simulink model "SimHA"  (R2022a)
settings: Solver=VariableStepAuto  StartTime=0.0  StopTime=20  RelTol=1e-3
values from neighbouring files (symbols this model uses):
  A = [4  0  0; 0  -9  0; 0  0  -1]    [HA1.mat]    (also in HA_1Matlabfile.m = [4 0 0; Home_assignment_1_Matlab_file.m = [4 0 0;0 -9 0;0 0 -1])
  B = [1  0; 1  0; 0  1]    [HA1.mat]    (also in HA_1Matlabfile.m = [1 0; Home_assignment_1_Matlab_file.m = [1 0;1 0;0 1])
  B1 = [1 1 0]    [HA1.mat]    (also in HA_1Matlabfile.m = [1; 1; 0]; Home_assignment_1_Matlab_file.m = [1;1;0])
  B2 = [0 0 1]    [HA1.mat]    (also in HA_1Matlabfile.m = [0; 0; 1]; Home_assignment_1_Matlab_file.m = [0;0;1])
  C = [-8  -9  1; 0  3  -3]    [HA1.mat]    (also in HA_1Matlabfile.m = [-8 -9 1; Home_assignment_1_Matlab_file.m = [-8 -9 1;0 3 -3])
  C1 = [-8 -9 -1]    [HA1.mat]    (also in HA_1Matlabfile.m = [-8 -9 1]; Home_assignment_1_Matlab_file.m)
  C2 = [0 3 -3]    [HA1.mat]    (also in HA_1Matlabfile.m; Home_assignment_1_Matlab_file.m)
  FV1 = [fv1 fv2 0]    [Home_assignment_1_Matlab_file.m]
  FV2 = [0 0 fv3]    [Home_assignment_1_Matlab_file.m]
  V1 = -3.36111388889    [HA1.mat]    (also in Home_assignment_1_Matlab_file.m = inv(-C1*inv(Abarr)*B1); Trial 1.m = inv(-C1*inv(Abarr)*B1); Trial1.m = inv(-C1*inv(Abarr)*B1))
  V2 = -3.66666666667    [HA1.mat]    (also in Home_assignment_1_Matlab_file.m = inv(-C2*inv(Abarr)*B2); Trial 1.m = inv(-C2*inv(Abarr)*B2); Trial1.m = inv(-C2*inv(Abarr)*B2))
settings Model: Creator=Abdur Rafay  LastModifiedBy=Abdur Rafay

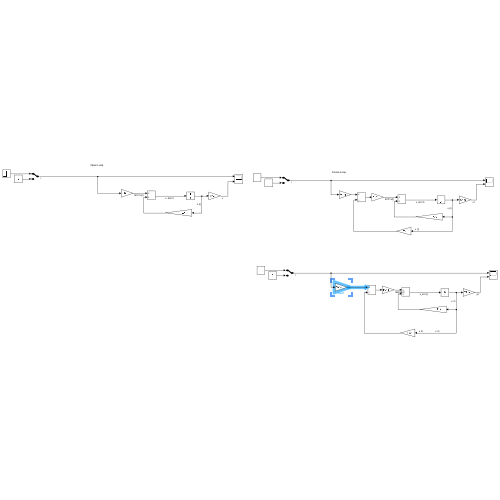
[thumbnail: Simulink's stored preview of the top-level diagram]
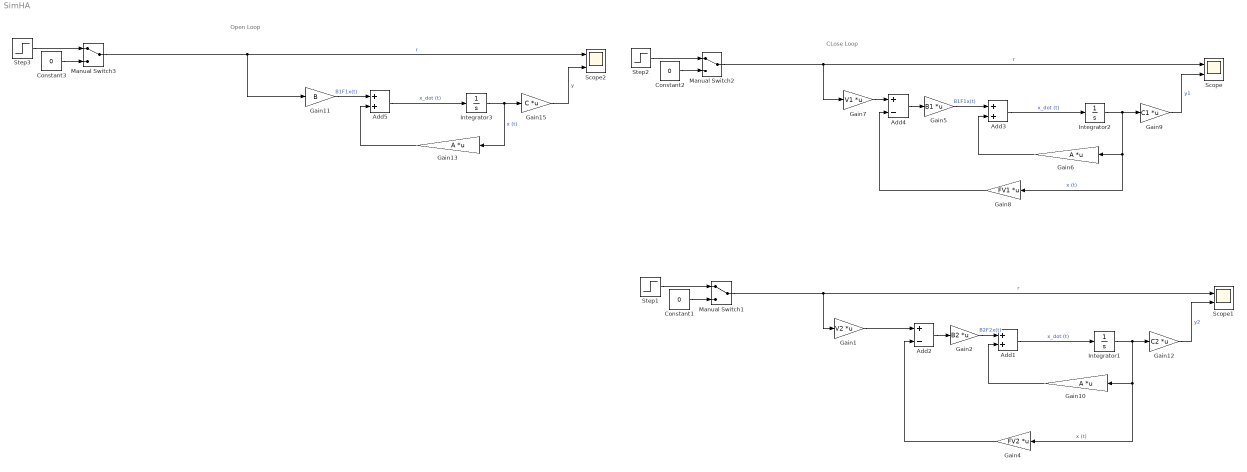
== system SimHA ==
  note: CLose Loop
  note: Open Loop
  Add1 : Sum
  Add2 : Sum  Inputs=+-
  Add3 : Sum
  Add4 : Sum  Inputs=+-
  Add5 : Sum
  Constant1 : Constant  Value=0
  Constant2 : Constant  Value=0
  Constant3 : Constant  Value=0
  Gain1 : Gain  Gain=V2  Multiplication=Matrix(K*u)
  Gain10 : Gain  Gain=A  Multiplication=Matrix(K*u)
  Gain11 : Gain  Gain=B
  Gain12 : Gain  Gain=C2  Multiplication=Matrix(K*u)
  Gain13 : Gain  Gain=A  Multiplication=Matrix(K*u)
  Gain15 : Gain  Gain=C  Multiplication=Matrix(K*u)
  Gain2 : Gain  Gain=B2  Multiplication=Matrix(K*u)
  Gain4 : Gain  Gain=FV2  Multiplication=Matrix(K*u)
  Gain5 : Gain  Gain=B1  Multiplication=Matrix(K*u)
  Gain6 : Gain  Gain=A  Multiplication=Matrix(K*u)
  Gain7 : Gain  Gain=V1  Multiplication=Matrix(K*u)
  Gain8 : Gain  Gain=FV1  Multiplication=Matrix(K*u)
  Gain9 : Gain  Gain=C1  Multiplication=Matrix(K*u)
  Integrator1 : Integrator
  Integrator2 : Integrator
  Integrator3 : Integrator
  Manual Switch1 : ManualSwitch
  Manual Switch2 : ManualSwitch
  Manual Switch3 : ManualSwitch
  Scope : Scope  NumInputPorts=2
  Scope1 : Scope  NumInputPorts=2
  Scope2 : Scope  NumInputPorts=2
  Step1 : Step  SampleTime=0
  Step2 : Step  SampleTime=0
  Step3 : Step  SampleTime=0
  wires:
  Integrator2/1 -> Gain9/1, Gain8/1, Gain6/1  "x (t)"
  Add3/1 -> Integrator2/1  "x_dot (t)"
  Gain6/1 -> Add3/2
  Add4/1 -> Gain5/1
  Step2/1 -> Manual Switch2/1
  Constant2/1 -> Manual Switch2/2
  Manual Switch2/1 -> Gain7/1, Scope/1  "r"
  Gain9/1 -> Scope/2  "y1"
  Gain12/1 -> Scope1/2  "y2"
  Step1/1 -> Manual Switch1/1
  Manual Switch1/1 -> Gain1/1, Scope1/1  "r"
  Add2/1 -> Gain2/1
  Gain10/1 -> Add1/2
  Add1/1 -> Integrator1/1  "x_dot (t)"
  Constant1/1 -> Manual Switch1/2
  Integrator1/1 -> Gain12/1, Gain4/1, Gain10/1  "x (t)"
  Gain1/1 -> Add2/1
  Gain5/1 -> Add3/1  "B1F1x(t)"
  Gain8/1 -> Add4/2
  Gain2/1 -> Add1/1  "B2F2x(t)"
  Gain4/1 -> Add2/2
  Gain11/1 -> Add5/1  "B1F1x(t)"
  Add5/1 -> Integrator3/1  "x_dot (t)"
  Step3/1 -> Manual Switch3/1
  Constant3/1 -> Manual Switch3/2
  Manual Switch3/1 -> Gain11/1, Scope2/1  "r"
  Integrator3/1 -> Gain13/1, Gain15/1  "x (t)"
  Gain13/1 -> Add5/2
  Gain15/1 -> Scope2/2  "y"
  Gain7/1 -> Add4/1
